simulink model "car1"  (Simulink 8.5)
settings: Solver=ode5  SolverMode=SingleTasking  StartTime=0.0  StopTime=45  FixedStep=0.01  MaxStep=0.01  RelTol=1e-3  AbsTol=1e-3
values from neighbouring files (symbols this model uses):
  b = Kf    (= 0.01)    [init.m]    (also in main.m)
  J = 0.02    [init.m]    (also in main.m)
  K = Kb    (= 0.1)    [init.m]    (also in main.m = place(A,B,[p1 p2]))
  L = 0.5    [init.m]    (also in main.m)
  R = 2.0    (= 2)    [init.m]    (also in main.m)
undefined symbols (not defined in the file): pidf_hw
settings Model: Creator=dsp520  LastModifiedBy=dsp520
settings DataIOCC: LimitDataPoints=off  SaveOutput=off  SaveTime=off
settings OptimizationCC: BlockReduction=off  BooleanDataType=off  ExpressionDepthLimit=128
settings DebuggingCC: SaveWithParameterizedLinksMsg=none  SignalResolutionControl=TryResolveAllWithWarning  MultiTaskDSMMsg=warning  MultiTaskCondExecSysMsg=none  FcnCallInpInsideContextMsg=EnableAllAsError  StateNameClashWarn=none  StrictBusMsg=None
settings HardwareCC: TargetUnknown=on
settings RTWCC: TemplateMakefile=grt_vc.tmf

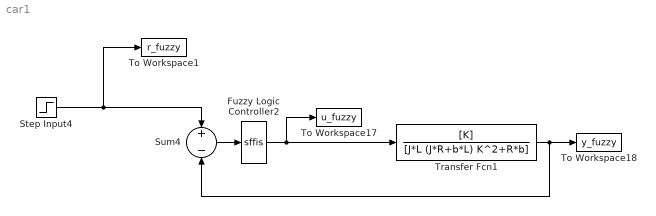
== system car1 ==
  Fuzzy Logic Controller2 : S-Function  FunctionName=sffis  Parameters=fismatrix  mask(FIS){fismatrix=pidf_hw}
      mask prompts: fismatrix "FIS Matrix:"
      mask help: FIS
      mask Help: Fuzzy Inference System
      mask Display: plot(0, -0.3, 6, -0.3, 0, 1.2, 6, 1.2, [0 6], [0 0], [1 2 3],[0 1 0],[2 3 4],[0 1 0],[3 4 5],[0 1 0])
  Step Input4 : Step  Time=0
  Sum4 : Sum  Inputs=+-  SaturateOnIntegerOverflow=on  InputSameDT=on  OutDataTypeStr=Inherit: Same as first input
  To Workspace1 : ToWorkspace  VariableName=r_fuzzy
      settings: MaxDataPoints=100000
  To Workspace17 : ToWorkspace  VariableName=u_fuzzy
      settings: MaxDataPoints=100000
  To Workspace18 : ToWorkspace  VariableName=y_fuzzy
      settings: MaxDataPoints=100000
  Transfer Fcn1 : TransferFcn  Numerator=[K]  Denominator=[J*L (J*R+b*L) K^2+R*b]
  wires:
  Fuzzy Logic Controller2/1 -> Transfer Fcn1/1, To Workspace17/1
  Sum4/1 -> Fuzzy Logic Controller2/1
  Transfer Fcn1/1 -> Sum4/2, To Workspace18/1
  Step Input4/1 -> To Workspace1/1, Sum4/1
